simulink model "first_order_system"  (R2023b)
settings: Solver=VariableStepAuto  StartTime=0.0  StopTime=10.0  MaxStep=1e-3  RelTol=1e-3
values from neighbouring files (symbols this model uses):
  k = 2    [Ramp_Function.m]    (also in Step_Function.m = 1)
  T = R*C    (= 0.001)    [Ramp_Function.m]    (also in Step_Function.m)
settings Model: Creator=hp  LastModifiedBy=hp

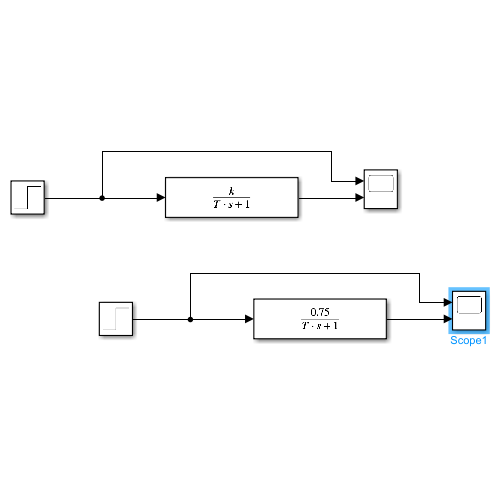
[thumbnail: Simulink's stored preview of the top-level diagram]
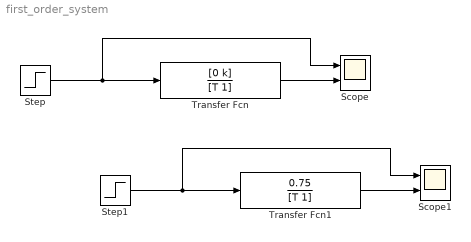
== system first_order_system ==
  Scope : Scope  NumInputPorts=2
  Scope1 : Scope  NumInputPorts=2
  Step : Step  SampleTime=0
  Step1 : Step  SampleTime=0
  Transfer Fcn : TransferFcn  Numerator=[0 k]  Denominator=[T 1]
  Transfer Fcn1 : TransferFcn  Numerator=[0 0.75]  Denominator=[T 1]
  wires:
  Step/1 -> Scope/1, Transfer Fcn/1
  Transfer Fcn/1 -> Scope/2
  Transfer Fcn1/1 -> Scope1/2
  Step1/1 -> Transfer Fcn1/1, Scope1/1
